simulink model "BF_sans_controleur"  (R2021b)
settings: Solver=VariableStepAuto  StartTime=0.0  StopTime=10.0  RelTol=1e-3
values from neighbouring files (symbols this model uses):
  A = [0 0 0  1 0 0   0 0 0   0 0 0 ... (first row only)    [systune_constant_gain_LPV.m]    (also in systune_gain_scheduling.m; systune_variable_gain_scheduling_LPV.m)
  B = diag([ws; chord; ws])    [external_force_moment.m]    (also in systune_constant_gain_LPV.m = [0 0 0 0; systune_gain_scheduling.m = [0 0 0 0; systune_variable_gain_scheduling_LPV.m = [0 0 0 0)
  B2 = [0 0 ... (first row only)    [systune_constant_gain_LPV.m]    (also in systune_gain_scheduling.m; systune_variable_gain_scheduling_LPV.m)
  C = [1 0 0 0 0 0 0 0 0 0 0 0 ... (144 elements, 12x12)]    [matrix.mat]    (also in matrix_lqr.mat = [1 0 0 0 0 0 0 0 0 0 0 0 ... (132 elements, 11x12)]; systune_constant_gain_LPV.m = eye(12); systune_gain_scheduling.m = eye(12); systune_variable_gain_scheduling_LPV.m = eye(12))
  C_control = [C(1:7,:);C(9:12,:)]    [systune_constant_gain_LPV.m]    (also in systune_gain_scheduling.m; systune_variable_gain_scheduling_LPV.m)
  D = q2dcm(q)    [external_force_moment.m]    (also in systune_constant_gain_LPV.m = zeros(12,6); systune_gain_scheduling.m = zeros(12,6); systune_variable_gain_scheduling_LPV.m = zeros(12,6))
  F = [1  0; 1  0; 0  1; 0  1]    [matrix.mat]    (also in matrix_lqr.mat; systune_constant_gain_LPV.m = [1 0; 1 0; 0 1; 0 1]; systune_gain_scheduling.m = [1 0; 1 0; 0 1; 0 1]; systune_variable_gain_scheduling_LPV.m = [1 0; 1 0; 0 1; 0 1])
  kw1 = 0.5    [systune_constant_gain_LPV.m]    (also in systune_gain_scheduling.m; systune_variable_gain_scheduling_LPV.m)
  kw2 = 10    [systune_constant_gain_LPV.m]    (also in systune_gain_scheduling.m; systune_variable_gain_scheduling_LPV.m)
  kw3 = 0.5    [systune_constant_gain_LPV.m]    (also in systune_gain_scheduling.m; systune_variable_gain_scheduling_LPV.m)
  x_12 = [[0; 0; 0]; [0; 0; 0]; [0; sin(angle/2); 0]; [0; 0; 0]]    [systune_constant_gain_LPV.m]    (also in systune_gain_scheduling.m; systune_variable_gain_scheduling_LPV.m)
settings Model: Creator=florian  LastModifiedBy=florian

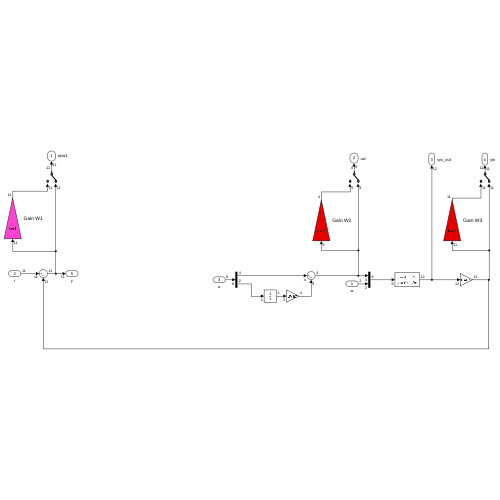
[thumbnail: Simulink's stored preview of the top-level diagram]
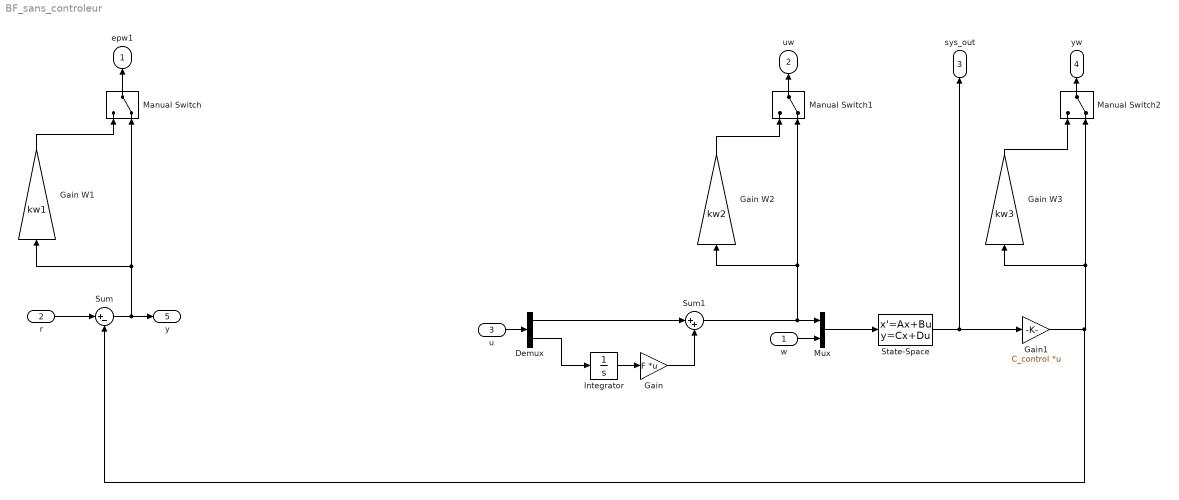
== system BF_sans_controleur ==
  w : Inport  PortDimensions=2
  r : Inport  Port=2  PortDimensions=11
  u : Inport  Port=3  PortDimensions=6
  Demux : Demux  Outputs=2
  Gain : Gain  Gain=F  Multiplication=Matrix(K*u) (u vector)
  Gain W1 : Gain  Gain=kw1  SaturateOnIntegerOverflow=on  OutDataTypeStr=Inherit: Same as input  ParamDataTypeStr=Inherit: Same as input
  Gain W2 : Gain  Gain=kw2  SaturateOnIntegerOverflow=on  OutDataTypeStr=Inherit: Same as input  ParamDataTypeStr=Inherit: Same as input
  Gain W3 : Gain  Gain=kw3  SaturateOnIntegerOverflow=on  OutDataTypeStr=Inherit: Same as input  ParamDataTypeStr=Inherit: Same as input
  Gain1 : Gain  Gain=C_control  Multiplication=Matrix(K*u) (u vector)
  Integrator : Integrator
  Manual Switch : ManualSwitch  CurrentSetting=0
  Manual Switch1 : ManualSwitch  CurrentSetting=0
  Manual Switch2 : ManualSwitch  CurrentSetting=0
  Mux : Mux  Inputs=2
  State-Space : StateSpace  A=A  B=[B, B2]  C=C  D=D  InitialCondition=x_12
  Sum : Sum  Inputs=|+-
  Sum1 : Sum  Inputs=|++
  epw1 : Outport  InitialOutput=0
  uw : Outport  Port=2  InitialOutput=0
  sys_out : Outport  Port=3  PortDimensions=12
  yw : Outport  Port=4  PortDimensions=11
  y : Outport  Port=5  PortDimensions=11
  wires:
  Mux/1 -> State-Space/1
  w/1 -> Mux/2
  r/1 -> Sum/1
  Sum/1 -> y/1, Gain W1/1, Manual Switch/2
  Sum1/1 -> Gain W2/1, Manual Switch1/2, Mux/1
  Manual Switch/1 -> epw1/1
  Gain W1/1 -> Manual Switch/1
  Manual Switch1/1 -> uw/1
  Gain W2/1 -> Manual Switch1/1
  State-Space/1 -> Gain1/1, sys_out/1
  u/1 -> Demux/1
  Demux/1 -> Sum1/1
  Gain/1 -> Sum1/2
  Integrator/1 -> Gain/1
  Demux/2 -> Integrator/1
  Gain1/1 -> Gain W3/1, Manual Switch2/2, Sum/2
  Manual Switch2/1 -> yw/1
  Gain W3/1 -> Manual Switch2/1
